simulink model "INTMRStEnCtrl"  (R2018b)
settings: Solver=FixedStepDiscrete  StartTime=0.0  StopTime=10.0  FixedStep=0.01  RelTol=1e-3
undefined symbols (not defined in the file or in its folder): data, SecRwLtStLtwdRtwdEn_Clear, SecRwLtStLtwdRtwdEn_Set, SecRwRtStFwdBkwdEn_Clear, SecRwRtStFwdBkwdEn_Set, SecRwRtStLtwdRtwdEn_Clear, SecRwRtStLtwdRtwdEn_Set
libraries: simulink x1
settings Model: Creator=sn2xws  LastModifiedBy=sn2xws
settings DataIOCC: SaveFormat=StructureWithTime
settings OptimizationCC: DefaultParameterBehavior=Inlined  EnhancedBackFolding=on  PassReuseOutputArgsAs=Individual arguments  ZeroExternalMemoryAtStartup=off  ZeroInternalMemoryAtStartup=off  OptimizeBlockOrder=speed  DifferentSizesBufferReuse=on  OptimizationCustomize=off
settings DebuggingCC: ParameterTunabilityLossMsg=error
settings ModelReferenceCC: ModelReferenceNumInstancesAllowed=Single
settings SFSimCC: MATLABDynamicMemAlloc=off
settings RTWCC: SystemTargetFile=autosar.tlc  GenCodeOnly=on  TemplateMakefile=ert_default_tmf  Description=AUTOSAR  GenerateReport=on  IncludeHyperlinkInReport=on  LaunchReport=on  GenerateTraceInfo=on  GenerateTraceReport=on  GenerateTraceReportSl=on  GenerateTraceReportSf=on  GenerateTraceReportEml=on  GenerateCodeMetricsReport=on
settings CodeAppCC: ForceParamTrailComments=on  IgnoreCustomStorageClasses=off  OperatorAnnotations=on  SimulinkDataObjDesc=on  SFDataObjDesc=on  InsertBlockDesc=on
settings STFCustomTargetCC: TargetLangStandard=C99 (ISO)  MultiwordLength=256  ParMdlRefBuildCompliant=on  CompOptLevelCompliant=on  IncludeMdlTerminateFcn=off  CombineOutputUpdateFcns=on  SuppressErrorStatus=on  ERTCustomFileBanners=on  SupportNonFinite=off  SupportComplex=off  SupportContinuousTime=off  SupportNonInlinedSFcns=off  RemoveResetFunc=on  MATLABClassNameForMDSCustomization=Simulink.SoftwareTarget.ERTCustomization  AutosarCompliant=on  UseToolchainInfoCompliant=on  LookupTableObjectStructAxisOrder=2,1,3,4,...  LUTObjectStructOrderEvenSpacing=Size,Table,Breakpoints  SystemTargetFile=autosar.tlc
settings ERTTargetCC: TargetLangStandard=C99 (ISO)  ConcurrentExecutionCompliant=off  IncludeMdlTerminateFcn=off  SuppressErrorStatus=on  SupportNonFinite=off  SupportComplex=off  ModelStepFunctionPrototypeControlCompliant=off  CPPClassGenCompliant=off  AutosarCompliant=on  LookupTableObjectStructAxisOrder=2,1,3,4,...  LUTObjectStructOrderEvenSpacing=Size,Table,Breakpoints  InlinedParameterPlacement=NonHierarchical  ERTCustomFileTemplate=example_file_process.tlc  ERTFilePackagingFormat=Compact

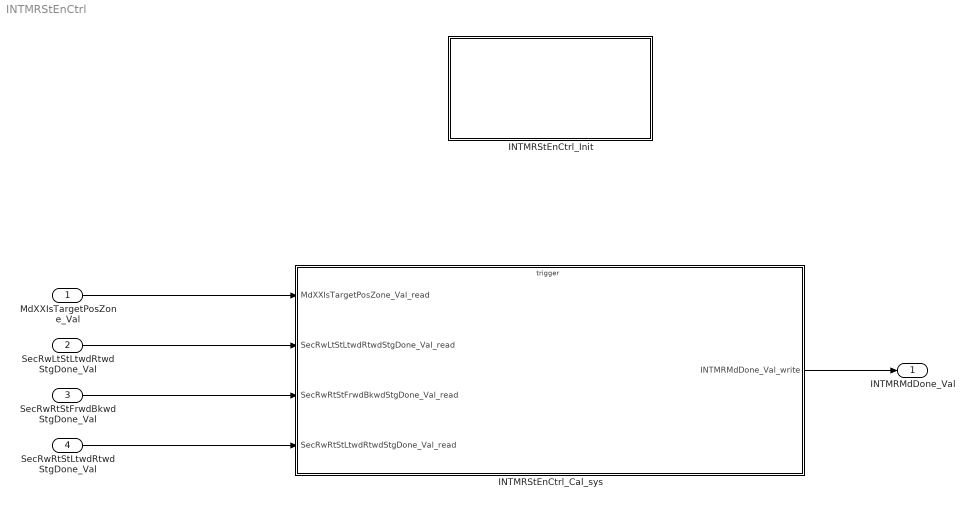
== system INTMRStEnCtrl ==
  MdXXIsTargetPosZone_Val : Inport  OutDataTypeStr=uint32  PortDimensions=1
  SecRwLtStLtwdRtwdStgDone_Val : Inport  Port=2  OutDataTypeStr=boolean  PortDimensions=1
  SecRwRtStFrwdBkwdStgDone_Val : Inport  Port=3  OutDataTypeStr=boolean  PortDimensions=1
  SecRwRtStLtwdRtwdStgDone_Val : Inport  Port=4  OutDataTypeStr=boolean  PortDimensions=1
  INTMRStEnCtrl_Cal_sys : Subsystem
  INTMRStEnCtrl_Init : Subsystem
  INTMRMdDone_Val : Outport  OutDataTypeStr=uint8  PortDimensions=1
  wires:
  MdXXIsTargetPosZone_Val/1 -> INTMRStEnCtrl_Cal_sys/1(MdXXIsTargetPosZone_Val_read)
  SecRwLtStLtwdRtwdStgDone_Val/1 -> INTMRStEnCtrl_Cal_sys/2(SecRwLtStLtwdRtwdStgDone_Val_read)
  SecRwRtStFrwdBkwdStgDone_Val/1 -> INTMRStEnCtrl_Cal_sys/3(SecRwRtStFrwdBkwdStgDone_Val_read)
  SecRwRtStLtwdRtwdStgDone_Val/1 -> INTMRStEnCtrl_Cal_sys/4(SecRwRtStLtwdRtwdStgDone_Val_read)
  INTMRStEnCtrl_Cal_sys/1(INTMRMdDone_Val_write) -> INTMRMdDone_Val/1

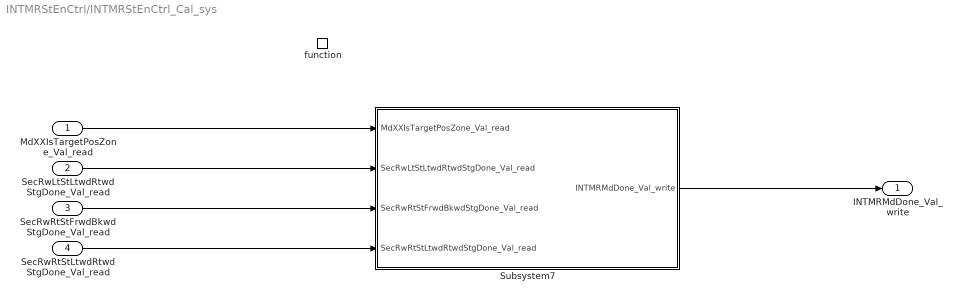
== system INTMRStEnCtrl/INTMRStEnCtrl_Cal_sys ==
  MdXXIsTargetPosZone_Val_read : Inport
  SecRwLtStLtwdRtwdStgDone_Val_read : Inport  Port=2
  SecRwRtStFrwdBkwdStgDone_Val_read : Inport  Port=3
  SecRwRtStLtwdRtwdStgDone_Val_read : Inport  Port=4
  function : TriggerPort  TriggerType=function-call  IsSimulinkFunction=on  FunctionName=INTMRStEnCtrl_Cal  VariantControl=(inherit)
  Subsystem7 : Subsystem
  INTMRMdDone_Val_write : Outport
      settings: EnsureOutportIsVirtual=on
  wires:
  Subsystem7/1(INTMRMdDone_Val_write) -> INTMRMdDone_Val_write/1
  MdXXIsTargetPosZone_Val_read/1 -> Subsystem7/1(MdXXIsTargetPosZone_Val_read)
  SecRwLtStLtwdRtwdStgDone_Val_read/1 -> Subsystem7/2(SecRwLtStLtwdRtwdStgDone_Val_read)
  SecRwRtStFrwdBkwdStgDone_Val_read/1 -> Subsystem7/3(SecRwRtStFrwdBkwdStgDone_Val_read)
  SecRwRtStLtwdRtwdStgDone_Val_read/1 -> Subsystem7/4(SecRwRtStLtwdRtwdStgDone_Val_read)

== system INTMRStEnCtrl/INTMRStEnCtrl_Init ==
  Event Listener : EventListener  EventName=reset

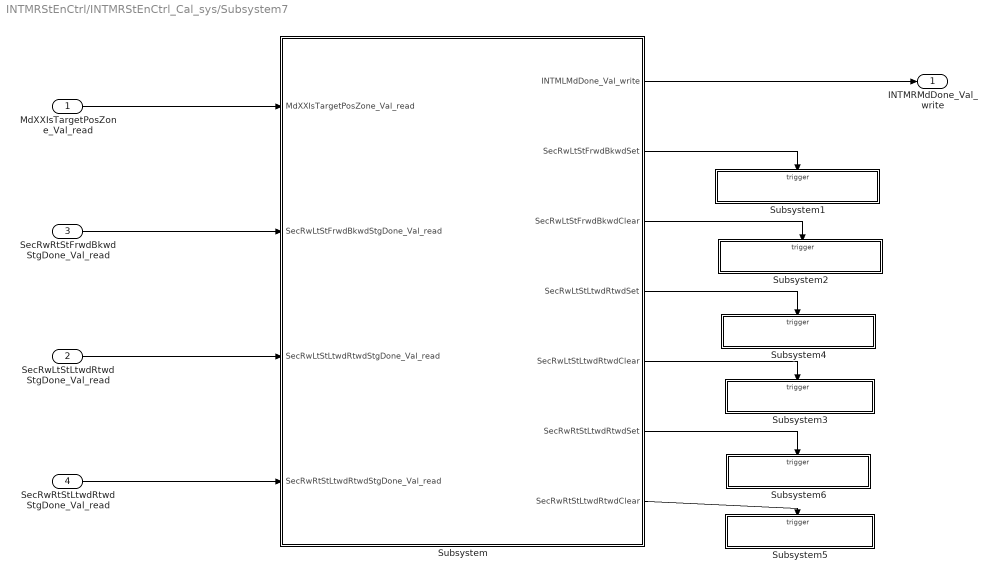
== system INTMRStEnCtrl/INTMRStEnCtrl_Cal_sys/Subsystem7 ==
  MdXXIsTargetPosZone_Val_read : Inport
  SecRwLtStLtwdRtwdStgDone_Val_read : Inport  Port=2
  SecRwRtStFrwdBkwdStgDone_Val_read : Inport  Port=3
  SecRwRtStLtwdRtwdStgDone_Val_read : Inport  Port=4
  Subsystem : Subsystem
  Subsystem1 : Subsystem
  Subsystem2 : Subsystem
  Subsystem3 : Subsystem
  Subsystem4 : Subsystem
  Subsystem5 : Subsystem
  Subsystem6 : Subsystem
  INTMRMdDone_Val_write : Outport
      settings: EnsureOutportIsVirtual=on
  wires:
  Subsystem/4(SecRwLtStLtwdRtwdSet) -> Subsystem4/Trigger
  Subsystem/5(SecRwLtStLtwdRtwdClear) -> Subsystem3/Trigger
  Subsystem/1(INTMLMdDone_Val_write) -> INTMRMdDone_Val_write/1
  SecRwRtStFrwdBkwdStgDone_Val_read/1 -> Subsystem/2(SecRwLtStFrwdBkwdStgDone_Val_read)
  Subsystem/2(SecRwLtStFrwdBkwdSet) -> Subsystem1/Trigger
  MdXXIsTargetPosZone_Val_read/1 -> Subsystem/1(MdXXIsTargetPosZone_Val_read)
  Subsystem/6(SecRwRtStLtwdRtwdSet) -> Subsystem6/Trigger
  SecRwLtStLtwdRtwdStgDone_Val_read/1 -> Subsystem/3(SecRwLtStLtwdRtwdStgDone_Val_read)
  SecRwRtStLtwdRtwdStgDone_Val_read/1 -> Subsystem/4(SecRwRtStLtwdRtwdStgDone_Val_read)
  Subsystem/3(SecRwLtStFrwdBkwdClear) -> Subsystem2/Trigger
  Subsystem/7(SecRwRtStLtwdRtwdClear) -> Subsystem5/Trigger

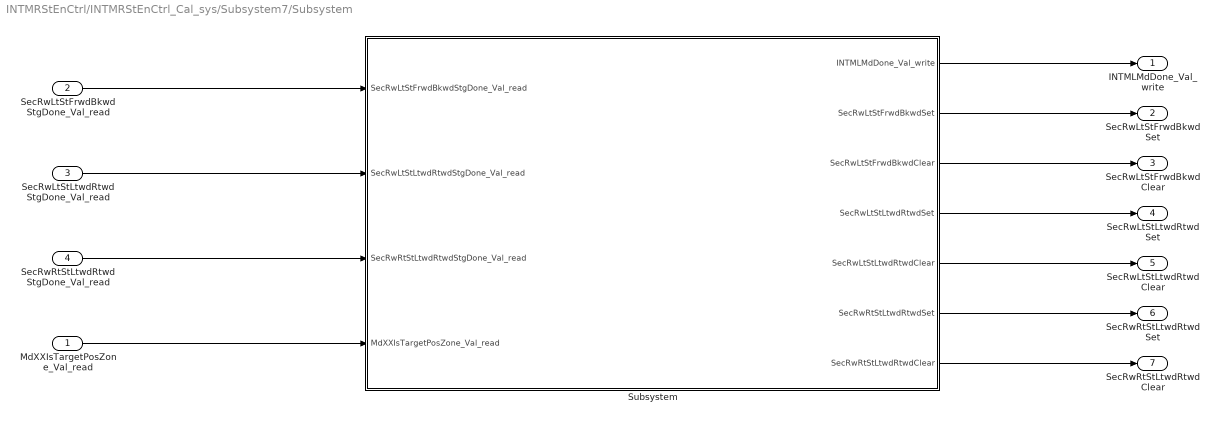
== system INTMRStEnCtrl/INTMRStEnCtrl_Cal_sys/Subsystem7/Subsystem ==
  MdXXIsTargetPosZone_Val_read : Inport
  SecRwLtStFrwdBkwdStgDone_Val_read : Inport  Port=2
  SecRwLtStLtwdRtwdStgDone_Val_read : Inport  Port=3
  SecRwRtStLtwdRtwdStgDone_Val_read : Inport  Port=4
  Subsystem : Subsystem
  INTMLMdDone_Val_write : Outport
      settings: EnsureOutportIsVirtual=on
  SecRwLtStFrwdBkwdSet : Outport  Port=2
  SecRwLtStFrwdBkwdClear : Outport  Port=3
  SecRwLtStLtwdRtwdSet : Outport  Port=4
  SecRwLtStLtwdRtwdClear : Outport  Port=5
  SecRwRtStLtwdRtwdSet : Outport  Port=6
  SecRwRtStLtwdRtwdClear : Outport  Port=7
  wires:
  Subsystem/1(INTMLMdDone_Val_write) -> INTMLMdDone_Val_write/1
  SecRwLtStFrwdBkwdStgDone_Val_read/1 -> Subsystem/1(SecRwLtStFrwdBkwdStgDone_Val_read)
  SecRwLtStLtwdRtwdStgDone_Val_read/1 -> Subsystem/2(SecRwLtStLtwdRtwdStgDone_Val_read)
  SecRwRtStLtwdRtwdStgDone_Val_read/1 -> Subsystem/3(SecRwRtStLtwdRtwdStgDone_Val_read)
  MdXXIsTargetPosZone_Val_read/1 -> Subsystem/4(MdXXIsTargetPosZone_Val_read)
  Subsystem/7(SecRwRtStLtwdRtwdClear) -> SecRwRtStLtwdRtwdClear/1
  Subsystem/6(SecRwRtStLtwdRtwdSet) -> SecRwRtStLtwdRtwdSet/1
  Subsystem/5(SecRwLtStLtwdRtwdClear) -> SecRwLtStLtwdRtwdClear/1
  Subsystem/3(SecRwLtStFrwdBkwdClear) -> SecRwLtStFrwdBkwdClear/1
  Subsystem/2(SecRwLtStFrwdBkwdSet) -> SecRwLtStFrwdBkwdSet/1
  Subsystem/4(SecRwLtStLtwdRtwdSet) -> SecRwLtStLtwdRtwdSet/1

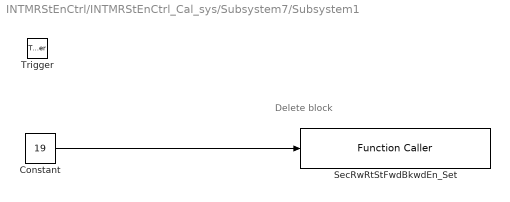
== system INTMRStEnCtrl/INTMRStEnCtrl_Cal_sys/Subsystem7/Subsystem1 ==
  note: Delete block
  Trigger : TriggerPort  TriggerType=function-call  VariantControl=Variant  PortDimensions=1
  Constant : Constant  Value=19  OutDataTypeStr=uint8
  SecRwRtStFwdBkwdEn_Set : FunctionCaller  FunctionPrototype=SecRwRtStFwdBkwdEn_Set(data)  InputArgumentSpecifications=uint8(1)
  wires:
  Constant/1 -> SecRwRtStFwdBkwdEn_Set/1

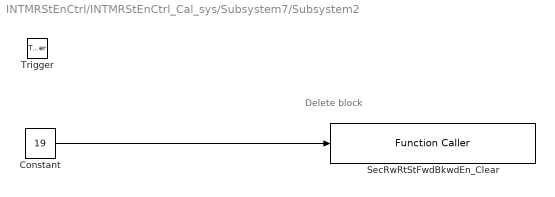
== system INTMRStEnCtrl/INTMRStEnCtrl_Cal_sys/Subsystem7/Subsystem2 ==
  note: Delete block
  Trigger : TriggerPort  TriggerType=function-call  VariantControl=Variant  PortDimensions=1
  Constant : Constant  Value=19  OutDataTypeStr=uint8
  SecRwRtStFwdBkwdEn_Clear : FunctionCaller  FunctionPrototype=SecRwRtStFwdBkwdEn_Clear(data)  InputArgumentSpecifications=uint8(1)
  wires:
  Constant/1 -> SecRwRtStFwdBkwdEn_Clear/1

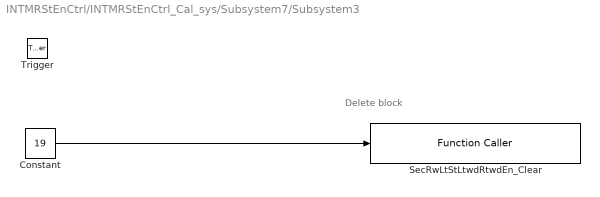
== system INTMRStEnCtrl/INTMRStEnCtrl_Cal_sys/Subsystem7/Subsystem3 ==
  note: Delete block
  Trigger : TriggerPort  TriggerType=function-call  VariantControl=Variant  PortDimensions=1
  Constant : Constant  Value=19  OutDataTypeStr=uint8
  SecRwLtStLtwdRtwdEn_Clear : FunctionCaller  FunctionPrototype=SecRwLtStLtwdRtwdEn_Clear(data)  InputArgumentSpecifications=uint8(1)
  wires:
  Constant/1 -> SecRwLtStLtwdRtwdEn_Clear/1

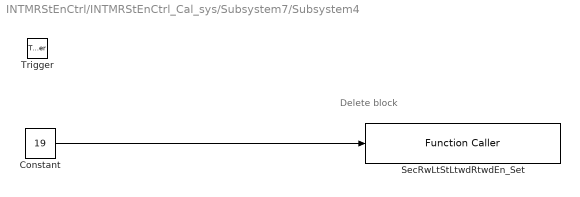
== system INTMRStEnCtrl/INTMRStEnCtrl_Cal_sys/Subsystem7/Subsystem4 ==
  note: Delete block
  Trigger : TriggerPort  TriggerType=function-call  VariantControl=Variant  PortDimensions=1
  Constant : Constant  Value=19  OutDataTypeStr=uint8
  SecRwLtStLtwdRtwdEn_Set : FunctionCaller  FunctionPrototype=SecRwLtStLtwdRtwdEn_Set(data)  InputArgumentSpecifications=uint8(1)
  wires:
  Constant/1 -> SecRwLtStLtwdRtwdEn_Set/1

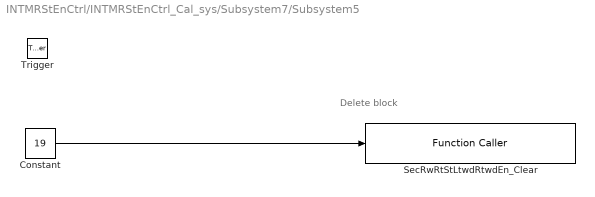
== system INTMRStEnCtrl/INTMRStEnCtrl_Cal_sys/Subsystem7/Subsystem5 ==
  note: Delete block
  Trigger : TriggerPort  TriggerType=function-call  VariantControl=Variant  PortDimensions=1
  Constant : Constant  Value=19  OutDataTypeStr=uint8
  SecRwRtStLtwdRtwdEn_Clear : FunctionCaller  FunctionPrototype=SecRwRtStLtwdRtwdEn_Clear(data)  InputArgumentSpecifications=uint8(1)
  wires:
  Constant/1 -> SecRwRtStLtwdRtwdEn_Clear/1

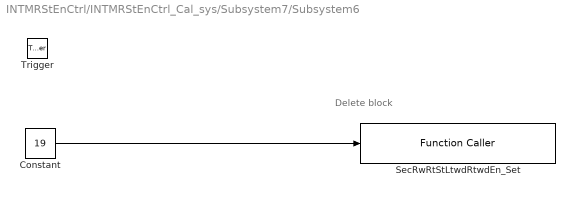
== system INTMRStEnCtrl/INTMRStEnCtrl_Cal_sys/Subsystem7/Subsystem6 ==
  note: Delete block
  Trigger : TriggerPort  TriggerType=function-call  VariantControl=Variant  PortDimensions=1
  Constant : Constant  Value=19  OutDataTypeStr=uint8
  SecRwRtStLtwdRtwdEn_Set : FunctionCaller  FunctionPrototype=SecRwRtStLtwdRtwdEn_Set(data)  InputArgumentSpecifications=uint8(1)
  wires:
  Constant/1 -> SecRwRtStLtwdRtwdEn_Set/1

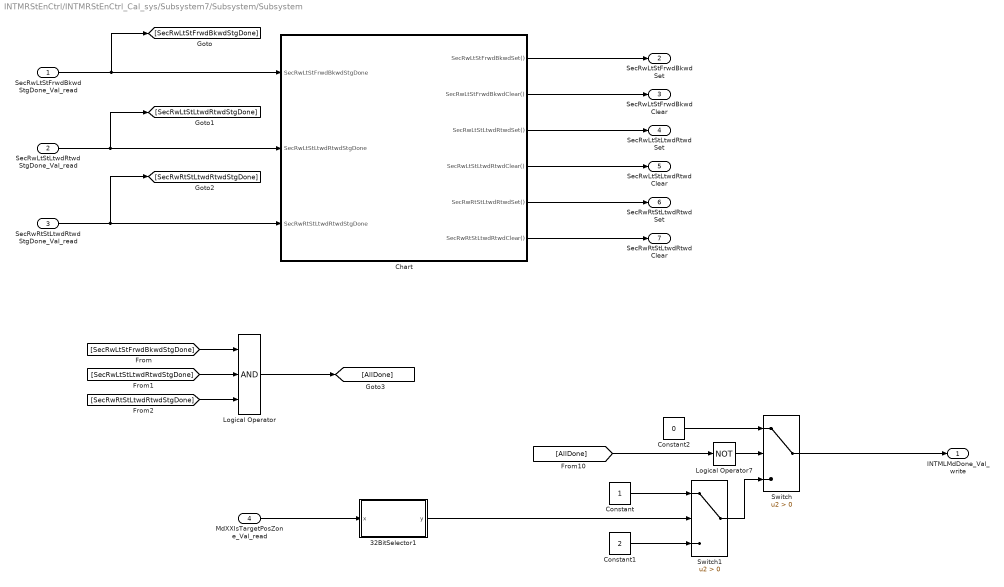
== system INTMRStEnCtrl/INTMRStEnCtrl_Cal_sys/Subsystem7/Subsystem/Subsystem ==
  SecRwLtStFrwdBkwdStgDone_Val_read : Inport
  SecRwLtStLtwdRtwdStgDone_Val_read : Inport  Port=2
  SecRwRtStLtwdRtwdStgDone_Val_read : Inport  Port=3
  MdXXIsTargetPosZone_Val_read : Inport  Port=4
  32BitSelector1 : Subsystem  mask(32 Bit Selector){BitNum=19}
      mask prompts: BitNum "Select Bit Number"
      mask help: Allows selection of a particular bit (0-31) out of a packed word up to 32 bits long. Output will be true if the bit number selected via the mask parameter is equal to one.
      mask TypeOptions BitNum: 0 | 1 | 2 | 3 | 4 | 5 | 6 | 7 | 8 | 9 | 10 | 11 | 12 | 13 | 14 | 15 | 16 | 17 | 18 | 19 | 20 | 21 | 22 | 23 | 24 | 25 | 26 | 27 | 28 | 29 | 30 | 31
      mask Display:
      | text(0.5, 0.8,'BIT','horizontalAlignment','center')
      | text(0.5, 0.5,'SELECTOR','horizontalAlignment','center')
      | text(0.5, 0.2,['-- Bit ',char(get_param(gcb,'BitNum')),' --'],'horizontalAlignment','center')
  Chart : Stateflow chart  TreatAsAtomicUnit=on
  Constant : Constant  OutDataTypeStr=uint8
  Constant1 : Constant  Value=2  OutDataTypeStr=uint8
  Constant2 : Constant  Value=0  OutDataTypeStr=uint8
  Logical Operator : Logic  Inputs=3  AllPortsSameDT=off  OutDataTypeStr=boolean
  Logical Operator7 : Logic  Operator=NOT  AllPortsSameDT=off  OutDataTypeStr=boolean
  Switch : Switch  Criteria=u2 > Threshold
  Switch1 : Switch  Criteria=u2 > Threshold
  INTMLMdDone_Val_write : Outport
      settings: EnsureOutportIsVirtual=on
  SecRwLtStFrwdBkwdSet : Outport  Port=2
  SecRwLtStFrwdBkwdClear : Outport  Port=3
  SecRwLtStLtwdRtwdSet : Outport  Port=4
  SecRwLtStLtwdRtwdClear : Outport  Port=5
  SecRwRtStLtwdRtwdSet : Outport  Port=6
  SecRwRtStLtwdRtwdClear : Outport  Port=7
  wires:
  Switch1/1 -> Switch/3
  MdXXIsTargetPosZone_Val_read/1 -> 32BitSelector1/1(x)
  Switch/1 -> INTMLMdDone_Val_write/1
  Chart/6(SecRwRtStLtwdRtwdClear()) -> SecRwRtStLtwdRtwdClear/1
  Chart/2(SecRwLtStFrwdBkwdClear()) -> SecRwLtStFrwdBkwdClear/1
  Chart/4(SecRwLtStLtwdRtwdClear()) -> SecRwLtStLtwdRtwdClear/1
  Chart/3(SecRwLtStLtwdRtwdSet()) -> SecRwLtStLtwdRtwdSet/1
  Chart/1(SecRwLtStFrwdBkwdSet()) -> SecRwLtStFrwdBkwdSet/1
  Chart/5(SecRwRtStLtwdRtwdSet()) -> SecRwRtStLtwdRtwdSet/1
  SecRwLtStLtwdRtwdStgDone_Val_read/1 -> [SecRwLtStLtwdRtwdStgDone], Chart/2(SecRwLtStLtwdRtwdStgDone)
  SecRwLtStFrwdBkwdStgDone_Val_read/1 -> [SecRwLtStFrwdBkwdStgDone], Chart/1(SecRwLtStFrwdBkwdStgDone)
  SecRwRtStLtwdRtwdStgDone_Val_read/1 -> [SecRwRtStLtwdRtwdStgDone], Chart/3(SecRwRtStLtwdRtwdStgDone)
  Logical Operator/1 -> [AllDone]
  [SecRwRtStLtwdRtwdStgDone] -> Logical Operator/3
  [SecRwLtStFrwdBkwdStgDone] -> Logical Operator/1
  [SecRwLtStLtwdRtwdStgDone] -> Logical Operator/2
  Constant2/1 -> Switch/1
  Constant1/1 -> Switch1/3
  Constant/1 -> Switch1/1
  Logical Operator7/1 -> Switch/2
  [AllDone] -> Logical Operator7/1
  32BitSelector1/1(y) -> Switch1/2

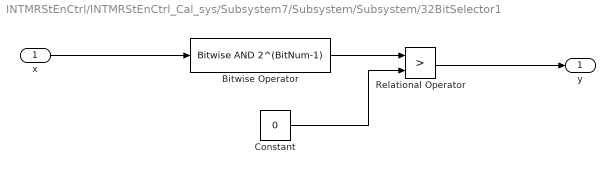
== system INTMRStEnCtrl/INTMRStEnCtrl_Cal_sys/Subsystem7/Subsystem/Subsystem/32BitSelector1 ==
  x : Inport
  Bitwise Operator : simulink/Logic and Bit Operations/Bitwise Operator  logicop=AND  UseBitMask=on  BitMask=2^(BitNum-1)  BitMaskRealWorld=Stored Integer
  Constant : Constant  Value=0  OutDataTypeStr=uint32
  Relational Operator : RelationalOperator  Operator=>  OutDataTypeStr=boolean  RndMeth=Simplest
  y : Outport
  wires:
  Relational Operator/1 -> y/1
  Constant/1 -> Relational Operator/2
  x/1 -> Bitwise Operator/1
  Bitwise Operator/1 -> Relational Operator/1

== stateflow chart INTMRStEnCtrl/INTMRStEnCtrl_Cal_sys/Subsystem7/Subsystem/Subsystem/Chart ==
  (default) -> (junction 9)
  (junction 9) -> (junction 49) [order 1] : [SecRwLtStFrwdBkwdStgDone]
  (junction 9) -> (junction 53) [order 2] : {
      | SecRwLtStFrwdBkwdSet;
      | }
  (junction 49) -> (junction 51) : {
      | SecRwLtStFrwdBkwdClear;
      | }
  (junction 51) -> (junction 53)
  (junction 53) -> (junction 121)
  (junction 121) -> (junction 122) [order 1] : [SecRwLtStLtwdRtwdStgDone]
  (junction 121) -> (junction 126) [order 2] : {
      | SecRwLtStLtwdRtwdSet;
      | }
  (junction 122) -> (junction 124) : {
      | SecRwLtStLtwdRtwdClear;
      | }
  (junction 124) -> (junction 126)
  (junction 126) -> (junction 60)
  (junction 60) -> (junction 62) [order 1] : [SecRwRtStLtwdRtwdStgDone]
  (junction 60) -> (junction 66) [order 2] : {
      | SecRwRtStLtwdRtwdSet;
      | }
  (junction 62) -> (junction 64) : {
      | SecRwRtStLtwdRtwdClear;
      | }
  (junction 64) -> (junction 66)
  data: SecRwLtStFrwdBkwdStgDone input boolean; SecRwLtStLtwdRtwdStgDone input boolean; SecRwRtStLtwdRtwdStgDone input boolean
  events: SecRwLtStFrwdBkwdSet output FUNCTION_CALL_EVENT; SecRwLtStFrwdBkwdClear output FUNCTION_CALL_EVENT; SecRwLtStLtwdRtwdSet output FUNCTION_CALL_EVENT; SecRwLtStLtwdRtwdClear output FUNCTION_CALL_EVENT; SecRwRtStLtwdRtwdSet output FUNCTION_CALL_EVENT; SecRwRtStLtwdRtwdClear output FUNCTION_CALL_EVENT
